simulink model "envMod"  (R2014b)
settings: Solver=ode1  StartTime=0.0  StopTime=10.0  FixedStep=0.01  RelTol=1e-3
settings Model: Creator=tramr  LastModifiedBy=tramr

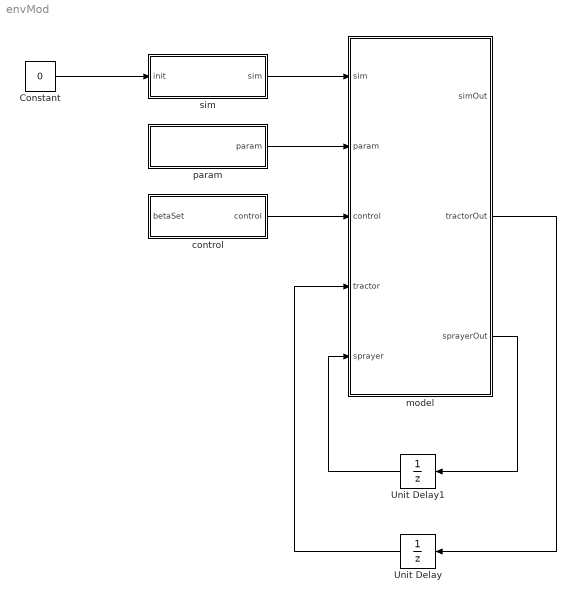
== system envMod ==
  Constant : Constant  Value=0  OutDataTypeStr=int16
  Unit Delay : UnitDelay  SampleTime=-1
  Unit Delay1 : UnitDelay  SampleTime=-1
  control : Subsystem
  model : MATLAB Function  TreatAsAtomicUnit=on
  param : Subsystem
  sim : Subsystem
  wires:
  sim/1(sim) -> model/1(sim)
  param/1(param) -> model/2(param)
  control/1(control) -> model/3(control)
  model/2(tractorOut) -> Unit Delay/1
  model/3(sprayerOut) -> Unit Delay1/1
  Unit Delay1/1 -> model/5(sprayer)
  Unit Delay/1 -> model/4(tractor)
  Constant/1 -> sim/1(init)

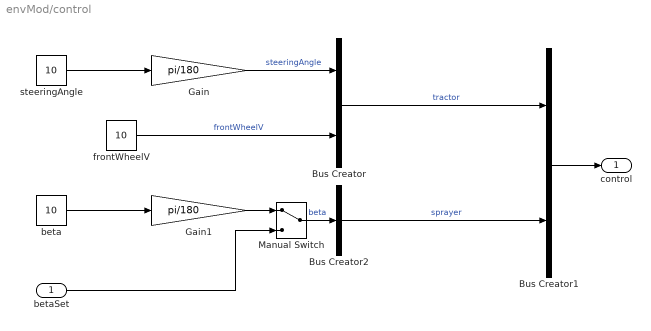
== system envMod/control ==
  betaSet : Inport
  Bus Creator : BusCreator  Inputs=2  OutDataTypeStr=Bus: controlTractorBusType
  Bus Creator1 : BusCreator  Inputs=2  OutDataTypeStr=Bus: controlBusType
  Bus Creator2 : BusCreator  Inputs=1  OutDataTypeStr=Bus: controlSprayerBusType
  Gain : Gain  Gain=pi/180
  Gain1 : Gain  Gain=pi/180
  Manual Switch : ManualSwitch
  beta : Constant  Value=10  OutDataTypeStr=double
  frontWheelV : Constant  Value=10  OutDataTypeStr=double
  steeringAngle : Constant  Value=10  OutDataTypeStr=double
  control : Outport
  wires:
  Bus Creator2/1 -> Bus Creator1/2  "sprayer"
  Bus Creator1/1 -> control/1
  Bus Creator/1 -> Bus Creator1/1  "tractor"
  steeringAngle/1 -> Gain/1
  Gain/1 -> Bus Creator/1  "steeringAngle"
  frontWheelV/1 -> Bus Creator/2  "frontWheelV"
  beta/1 -> Gain1/1
  Manual Switch/1 -> Bus Creator2/1  "beta"
  Gain1/1 -> Manual Switch/1
  betaSet/1 -> Manual Switch/2

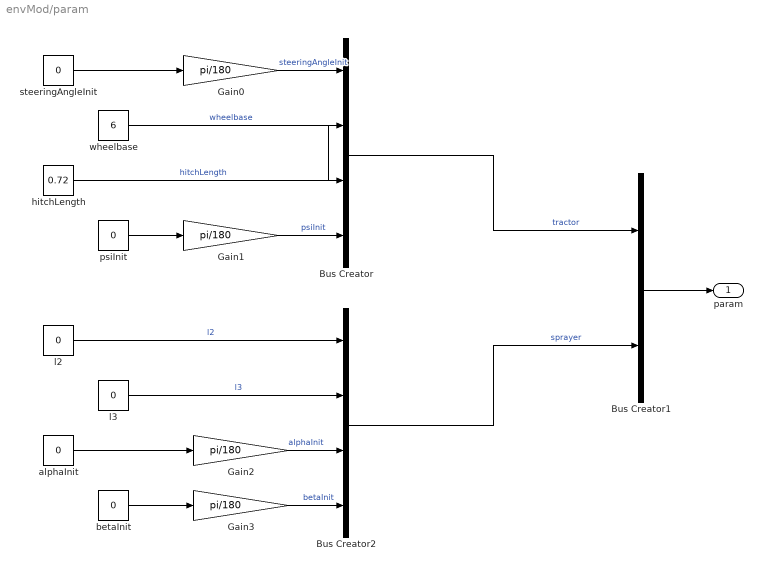
== system envMod/param ==
  Bus Creator : BusCreator  OutDataTypeStr=Bus: paramTractorBusType
  Bus Creator1 : BusCreator  Inputs=2  OutDataTypeStr=Bus: paramBusType
  Bus Creator2 : BusCreator  OutDataTypeStr=Bus: paramSprayerBusType
  Gain{0..3} (4 alike) : Gain  Gain=pi/180
  alphaInit : Constant  Value=0  OutDataTypeStr=double
  betaInit : Constant  Value=0  OutDataTypeStr=double
  hitchLength : Constant  Value=0.72  OutDataTypeStr=double
  l2 : Constant  Value=0  OutDataTypeStr=double
  l3 : Constant  Value=0  OutDataTypeStr=double
  psiInit : Constant  Value=0  OutDataTypeStr=double
  steeringAngleInit : Constant  Value=0  OutDataTypeStr=double
  wheelbase : Constant  Value=6  OutDataTypeStr=double
  param : Outport
  wires:
  steeringAngleInit/1 -> Gain0/1
  wheelbase/1 -> Bus Creator/3  "wheelbase"
  Bus Creator/1 -> Bus Creator1/1  "tractor"
  Bus Creator1/1 -> param/1
  Bus Creator2/1 -> Bus Creator1/2  "sprayer"
  hitchLength/1 -> Bus Creator/2  "hitchLength"
  psiInit/1 -> Gain1/1
  Gain1/1 -> Bus Creator/4  "psiInit"
  l2/1 -> Bus Creator2/1  "l2"
  l3/1 -> Bus Creator2/2  "l3"
  betaInit/1 -> Gain3/1
  alphaInit/1 -> Gain2/1
  Gain2/1 -> Bus Creator2/3  "alphaInit"
  Gain3/1 -> Bus Creator2/4  "betaInit"
  Gain0/1 -> Bus Creator/1  "steeringAngleInit"

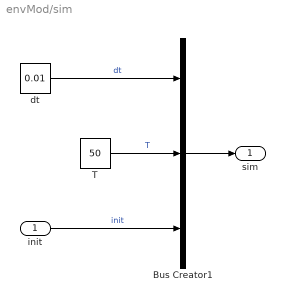
== system envMod/sim ==
  init : Inport  OutDataTypeStr=int16
  Bus Creator1 : BusCreator  Inputs=3  OutDataTypeStr=Bus: simBusType
  T : Constant  Value=50  OutDataTypeStr=int16
  dt : Constant  Value=0.01  OutDataTypeStr=int16
  sim : Outport
  wires:
  Bus Creator1/1 -> sim/1
  dt/1 -> Bus Creator1/1  "dt"
  T/1 -> Bus Creator1/2  "T"
  init/1 -> Bus Creator1/3  "init"

== matlab function envMod/model ==
  data: simOut output Bus: simBusType; sim input Bus: simBusType; param input Bus: paramBusType; tractorOut output Bus: tractorBusType; control input Bus: controlBusType; tractor input Bus: tractorBusType; sprayer input Bus: sprayerBusType; sprayerOut output Bus: sprayerBusType
function [simOut, tractorOut, sprayerOut] = model(sim, param, control, tractor, sprayer)
    if (sim.init == 0)
        simOut.init                = (int16)1;
        
        % tractor
        tractorOut.frontX          = 0;
        tractorOut.frontY          = 0;

        tractorOut.rearX           = tractor.frontX - ...
                                  param.tractor.wheelbase * ...
                                  cos(param.tractor.psiInit);
        tractorOut.rearY           = tractor.frontY - ...
                                  param.tractor.wheelbase * ...
                                  sin(param.tractor.psiInit);


        tractorOut.hitchX          = tractor.rearX - ...
                                  param.tractor.hitchLength * ...
                                  cos(param.tractor.psiInit);
        tractorOut.hitchY          = tractor.rearY - ...
                                  param.tractor.hitchLength * ...
                                  sin(param.tractor.psiInit);

        tractorOut.psi             = tan(...
                                  (tractor.frontY - tractor.rearY)/...
                                  (tractor.frontX - tractor.rearX));


        % sprayer
        sprayerOut.hitchX          = tractor.hitchX;

        sprayerOut.hitchY          = tractor.hitchY;

        sprayerOut.kinkX           = sprayer.hitchX - ...
                                  param.sprayer.l2 * ...
                                  cos(param.tractor.psiInit + param.sprayer.alphaInit);

        sprayerOut.kinkY           = sprayer.hitchY - ...
                                  param.sprayer.l2 * ...
                                  sin(param.tractor.psiInit + param.sprayer.alphaInit);

        sprayerOut.axisX           = sprayer.kinkX - ...
                                  param.sprayer.l3 * ...
                                  cos(param.tractor.psiInit + param.sprayer.alphaInit + param.sprayer.betaInit);

        sprayerOut.axisY           = sprayer.kinkY - ...
                                  param.sprayer.l3 * ...
                                  sin(param.tractor.psiInit + param.sprayer.alphaInit + param.sprayer.betaInit);

        sprayerOut.alpha           = param.sprayer.alphaInit;
                              
        sprayerOut.psi             = tan(...
                                  (sprayer.hitchY - sprayer.kinkY)/...
                                  (sprayer.hitchX - sprayer.kinkX));

        sprayerOut.dpsi            = 0;

        sprayerOut.ds              = 0;


        
    else
        %% helper
        deltaS = control.tractor.frontWheelV * sim.dt;

        dPsiTractor = asin(deltaS * sin(pi - control.tractor.steeringAngle) / param.tractor.wheelbase);

        %% calculation

        % tractor

        tractor.psi = tractor.psi + dPsiTractor;

        if (tractor.psi >  pi)
            tractor.psi = tractor.psi - 2*pi;
        end

        if (tractor.psi < -pi)
            tractor.psi = tractor.psi + 2*pi;
        end

        %front
        tractor.frontX = tractor.frontX + ...
                         deltaS * cos(control.tractor.steeringAngle + tractor.psi);

        tractor.frontY = tractor.frontY + ...
                         deltaS * sin(control.tractor.steeringAngle + tractor.psi);

        % rear
        tractor.rearX = tractor.frontX - ...
                        param.tractor.wheelbase * ...
                        cos(tractor.psi);
        tractor.rearY = tractor.frontY - ...
                        param.tractor.wheelbase * ...
                        sin(tractor.psi);

        % hitch
        tractor.hitchX = tractor.rearX - ...
                         param.tractor.hitchLength * ...
                         cos(tractor.psi);
        tractor.hitchY = tractor.rearY - ...
                         param.tractor.hitchLength * ...
                         sin(tractor.psi);

        % sprayer

        psiSprayerOld = sprayer.psi;
        axisXSprayerOld = sprayer.axisX;
        axisYSprayerOld = sprayer.axisY;

        % diagonal plane between old axis and old hitch position
        diagSprayer = sqrt(param.sprayer.l2^2 + param.sprayer.l3^2 ...
                           - 2 * param.sprayer.l2 * param.sprayer.l3 ...
                           * cos(pi - control.sprayer.beta));

        tau1 =  epsCheck(asin(param.sprayer.l3 * sin(pi - control.sprayer.beta) / diagSprayer));
        tau2 =  epsCheck(asin(param.sprayer.l2 * sin(pi - control.sprayer.beta) / diagSprayer));

        % straight through kink (kinkX, kinkX) and axis (axisX, axisY)
        if (param.sprayer.l3 == 0)
            % l3 == 0 (wheelsteer)
            A = [sprayer.kinkX 1; sprayer.kinkX + cos(sprayer.psi + control.sprayer.beta) 1];
            b = [sprayer.kinkY  ; sprayer.kinkY + sin(sprayer.psi + control.sprayer.beta)  ];

            result = A\b;       % solving the linear system

            m = result(1);      % slope
            c = result(2);      % y-intercept
        else
            % l3 > 0
            A = [sprayer.kinkX 1; sprayer.axisX 1];
            b = [sprayer.kinkY  ; sprayer.axisY  ];

            result = A\b;       % solving the linear system

            m = result(1);      % slope
            c = result(2);      % y-intercept
        end



        % cycle with hitch_new as center (hitchX, hitchY) and radius diagSprayer
        % formula: (x - x0)^2 + (y - y0)^2 = r^2
        x(1) = (tractor.hitchX + (- c^2 - 2*c*tractor.hitchX*m + 2*c*tractor.hitchY - tractor.hitchX^2*m^2 + 2*tractor.hitchX*tractor.hitchY*m - tractor.hitchY^2 + m^2*diagSprayer^2 + diagSprayer^2)^(1/2) - c*m + tractor.hitchY*m)/(m^2 + 1);
        x(2) = (tractor.hitchX - (- c^2 - 2*c*tractor.hitchX*m + 2*c*tractor.hitchY - tractor.hitchX^2*m^2 + 2*tractor.hitchX*tractor.hitchY*m - tractor.hitchY^2 + m^2*diagSprayer^2 + diagSprayer^2)^(1/2) - c*m + tractor.hitchY*m)/(m^2 + 1);

        y(1) = (c + tractor.hitchX*m + tractor.hitchY*m^2 + m*(- c^2 - 2*c*tractor.hitchX*m + 2*c*tractor.hitchY - tractor.hitchX^2*m^2 + 2*tractor.hitchX*tractor.hitchY*m - tractor.hitchY^2 + m^2*diagSprayer^2 + diagSprayer^2)^(1/2))/(m^2 + 1);
        y(2) = (c + tractor.hitchX*m + tractor.hitchY*m^2 - m*(- c^2 - 2*c*tractor.hitchX*m + 2*c*tractor.hitchY - tractor.hitchX^2*m^2 + 2*tractor.hitchX*tractor.hitchY*m - tractor.hitchY^2 + m^2*diagSprayer^2 + diagSprayer^2)^(1/2))/(m^2 + 1);

        if (sqrt(abs(sprayer.axisX - x(1))^2 + abs(sprayer.axisY - y(1))^2) < ...
            sqrt(abs(sprayer.axisX - x(2))^2 + abs(sprayer.axisY - y(2))^2))

            sprayer.axisX = x(1);
            sprayer.axisY = y(1);
        else
            sprayer.axisX = x(2);
            sprayer.axisY = y(2);
        end

        sprayer.hitchX = tractor.hitchX;
        sprayer.hitchY = tractor.hitchY;

        diagAngle = atan2((sprayer.hitchY - sprayer.axisY) , ...
                          (sprayer.hitchX - sprayer.axisX));

        sprayer.kinkX = sprayer.hitchX - param.sprayer.l2 * cos(diagAngle - tau1);
        sprayer.kinkY = sprayer.hitchY - param.sprayer.l2 * sin(diagAngle - tau1);

        if (param.sprayer.l3 == 0)
            sprayer.psi = diagAngle;
        else
            sprayer.psi = atan((sprayer.axisY - sprayer.kinkY) / ...
                               (sprayer.axisX - sprayer.kinkX));
        end

        sprayer.alpha = -(tractor.psi - sprayer.psi);

        if sprayer.alpha < -pi
            sprayer.alpha = sprayer.alpha + 2*pi;
        end
        if sprayer.alpha >  pi
            sprayer.alpha = sprayer.alpha - 2*pi;
        end


        sprayer.dpsi = mod(psiSprayerOld - sprayer.psi, pi);

        sprayer.ds = sqrt((axisXSprayerOld - sprayer.axisX)^2 + ...
                          (axisYSprayerOld - sprayer.axisY)^2);

        %% set outputs
        tractorOut  = tractor;
        sprayerOut  = sprayer;
    end
end
